simulink model "Es2_simulink"  (R2023a)
settings: Solver=VariableStepAuto  StartTime=0.0  StopTime=30  RelTol=1e-3
undefined symbols (not defined in the file or in its folder): ES2_emg, fdesignblkfcn, gcbh
libraries: dspfdesign x4, vrlib x1
settings Model: Creator=pisy1  LastModifiedBy=pisy1

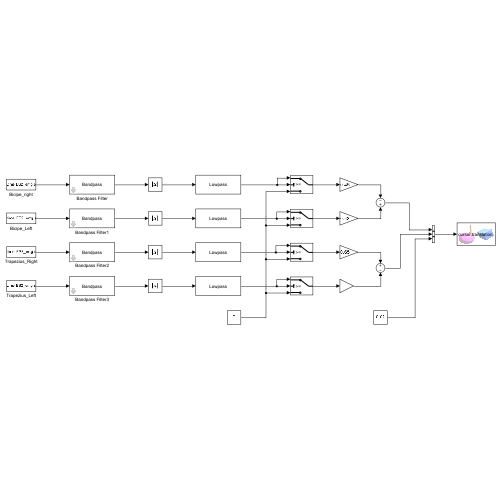
[thumbnail: Simulink's stored preview of the top-level diagram]
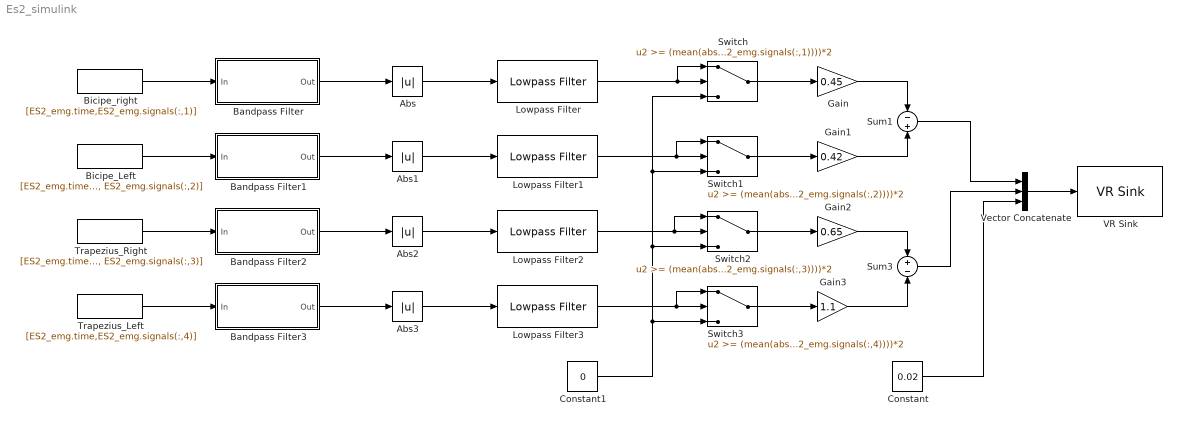
== system Es2_simulink ==
  Abs{,1..3} (4 alike) : Abs  SaturateOnIntegerOverflow=off
  Bandpass Filter : Subsystem  DialogController=fdesignblkfcn  InitFcn=fdesignblkfcn(gcbh, {'InitFcn'});  mask(Bandpass Filter){}
      mask help: dsp:DSPFilterDesignBlockDialog:BandpassFdesign_MaskDesc
      settings: CopyFcn=fdesignblkfcn(gcbh, {'CopyFcn'});
      mask Help: helpview(mapfilelocation('dsp'), 'dspbandpassfilter');
      mask Display: disp('Bandpass');
  Bandpass Filter1 : Subsystem  DialogController=fdesignblkfcn  InitFcn=fdesignblkfcn(gcbh, {'InitFcn'});  mask(Bandpass Filter){}
      mask help: dsp:DSPFilterDesignBlockDialog:BandpassFdesign_MaskDesc
      settings: CopyFcn=fdesignblkfcn(gcbh, {'CopyFcn'});
      mask Help: helpview(mapfilelocation('dsp'), 'dspbandpassfilter');
      mask Display: disp('Bandpass');
  Bandpass Filter2 : Subsystem  DialogController=fdesignblkfcn  InitFcn=fdesignblkfcn(gcbh, {'InitFcn'});  mask(Bandpass Filter){}
      mask help: dsp:DSPFilterDesignBlockDialog:BandpassFdesign_MaskDesc
      settings: CopyFcn=fdesignblkfcn(gcbh, {'CopyFcn'});
      mask Help: helpview(mapfilelocation('dsp'), 'dspbandpassfilter');
      mask Display: disp('Bandpass');
  Bandpass Filter3 : Subsystem  DialogController=fdesignblkfcn  InitFcn=fdesignblkfcn(gcbh, {'InitFcn'});  mask(Bandpass Filter){}
      mask help: dsp:DSPFilterDesignBlockDialog:BandpassFdesign_MaskDesc
      settings: CopyFcn=fdesignblkfcn(gcbh, {'CopyFcn'});
      mask Help: helpview(mapfilelocation('dsp'), 'dspbandpassfilter');
      mask Display: disp('Bandpass');
  Bicipe_Left : FromWorkspace  VariableName=[ES2_emg.time, ES2_emg.signals(:,2)]  SampleTime=1/1000
  Bicipe_right : FromWorkspace  VariableName=[ES2_emg.time,ES2_emg.signals(:,1)]  SampleTime=1/1000
  Constant : Constant  Value=0.02
  Constant1 : Constant  Value=0
  Gain : Gain  Gain=0.45
  Gain1 : Gain  Gain=0.42
  Gain2 : Gain  Gain=0.65
  Gain3 : Gain  Gain=1.1
  Lowpass Filter{,1..3} (4 alike) : dspfdesign/Lowpass Filter  FilterType=FIR  DesignForMinimumOrder=on  FilterOrder=50  PassbandFrequency=3  StopbandFrequency=6  PassbandRipple=0.1  StopbandAttenuation=80  SampleRateMode=Specify on dialog  SampleRate=1000  SimulateUsing=Interpreted execution  roundingMode=Floor  coeffsDataTypeStr=fixdt(1,16)
  Sum1 : Sum  Inputs=-|+
  Sum3 : Sum  Inputs=+|-
  Switch : Switch  Threshold=(mean(abs(ES2_emg.signals(:,1))))*2  SaturateOnIntegerOverflow=off  InputSameDT=off
  Switch1 : Switch  Threshold=(mean(abs(ES2_emg.signals(:,2))))*2  SaturateOnIntegerOverflow=off  InputSameDT=off
  Switch2 : Switch  Threshold=(mean(abs(ES2_emg.signals(:,3))))*2  SaturateOnIntegerOverflow=off  InputSameDT=off
  Switch3 : Switch  Threshold=(mean(abs(ES2_emg.signals(:,4))))*2  SaturateOnIntegerOverflow=off  InputSameDT=off
  Trapezius_Left : FromWorkspace  VariableName=[ES2_emg.time,ES2_emg.signals(:,4)]  SampleTime=1/1000
  Trapezius_Right : FromWorkspace  VariableName=[ES2_emg.time, ES2_emg.signals(:,3)]  SampleTime=1/1000
  VR Sink : vrlib/VR Sink  InstantiateOnLoad=on  SampleTime=0.1  ViewEnable=on  RemoteChange=off  RemoteView=off  FieldsWritten=cursor.translation.3.1.1.double  WorldFileName=8_palline_color.wrl  AutoView=off  VideoDimensions=[]  AllowVariableSize=off
  Vector Concatenate : Concatenate  NumInputs=3
  wires:
  Bandpass Filter/1(Out) -> Abs/1
  Abs/1 -> Lowpass Filter/1
  Abs1/1 -> Lowpass Filter1/1
  Abs2/1 -> Lowpass Filter2/1
  Abs3/1 -> Lowpass Filter3/1
  Bandpass Filter3/1(Out) -> Abs3/1
  Bandpass Filter2/1(Out) -> Abs2/1
  Bandpass Filter1/1(Out) -> Abs1/1
  Constant/1 -> Vector Concatenate/3
  Constant1/1 -> Switch/3, Switch1/3, Switch2/3, Switch3/3
  Lowpass Filter/1 -> Switch/1, Switch/2
  Lowpass Filter1/1 -> Switch1/1, Switch1/2
  Lowpass Filter2/1 -> Switch2/1, Switch2/2
  Lowpass Filter3/1 -> Switch3/1, Switch3/2
  Vector Concatenate/1 -> VR Sink/1
  Sum1/1 -> Vector Concatenate/1
  Sum3/1 -> Vector Concatenate/2
  Switch3/1 -> Gain3/1
  Switch2/1 -> Gain2/1
  Switch1/1 -> Gain1/1
  Switch/1 -> Gain/1
  Bicipe_Left/1 -> Bandpass Filter1/1(In)
  Bicipe_right/1 -> Bandpass Filter/1(In)
  Trapezius_Left/1 -> Bandpass Filter3/1(In)
  Trapezius_Right/1 -> Bandpass Filter2/1(In)
  Gain/1 -> Sum1/1
  Gain3/1 -> Sum3/2
  Gain2/1 -> Sum3/1
  Gain1/1 -> Sum1/2

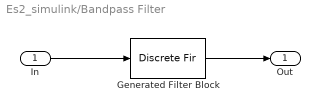
== system Es2_simulink/Bandpass Filter ==
  In : Inport
  Generated Filter Block : DiscreteFir  Tag=BlockMethodSubSystem  Coefficients=[-0.00268732969538467564 -0.0118693634414288839 -0.00464956295920984381 0.0192244660845699369 0.00401606132782830055 0.00113331359240486512 0.0081600274662763702 -0.00337347421316901196 0.00485232718819333594 -0.00260504936894014657 0.000574747267355126337 -0.00105940036214936546 -0.00260380481464203214 -1.31551187216019314e-05 -0.00436007271689453288 0.000301810052777536694 -0.00481839310143463047 -4.27651908615003795e-05 -0.00419699330761031525 -0.000850466496812417837 -0.002776431768186669 -0.00183710618674402196 -0.000931746391162900471 -0.00263535219191951726 0.000919518489321216603 -0.00287750193371332213 0.00234181011288215127 -0.0022885925310662655 0.00303033934142757019 -0.000818319173867537199 0.00290108759067781666 0.00132279014325093619 0.00211108519395160864 0.00367085202435546605 0.00104360943564956506 0.00558442951144205377 0.000169105346465872608 0.00645654583445923191 -0.000119621272358262989 0.00588287758558112082 0.000336400896954254514 0.00385123203778863117 0.00136139168005587272 0.000749506211944570011 0.00246191925777084104 -0.00266439972783858933 0.00298201898694502344 -0.0055265059231050977 0.00236131888729237136 -0.00708353416263684393 0.00033450104078665624 -0.00696088627834120025 -0.00288568812972243328 -0.0052797356224147194 -0.0065775442931197952 -0.00268218418692768058 -0.00964697208745706782 -7.2233731547276421e-05 -0.0109531527675894441 0.0016467062272919929 -0.00970504643296686217 0.00193564453488831792 -0.00571167618718560616 0.000850667168220128195 0.000409739809056720167 -0.000946605415802572597 0.00733164384418515808 -0.00232570671431918917 0.0133293503468598154 -0.00208261382497140855 0.0167413845912259031 0.000543802062682958998 0.0165183040724974223 0.00555728090932838467 0.0126095283934480155 0.0119157946244619097 0.00590275310015039509 0.0176861788427832844 -0.00170987438306957965 0.0205602710112455442 -0.0080752621768838441 0.0182809523079280126 -0.0113873648721023804 0.00965729454439472057 -0.0108374323953576782 -0.00513335134094568962 -0.00697642486247677246 -0.0240941247073598527 -0.00194247899233986054 -0.0437115227268439765 0.000972484332068239681 -0.0593855417670438313 -0.00220178639407756643 -0.0661386206551100586 -0.0155029767222636811 -0.0588085413080414038 -0.0436952688973444303 -0.0302190186977819297 -0.0973608444785738353 0.0433085287546407308 -0.244561056960632628 0.576859281938552626 0.576859281938552626 -0.244561056960632628 0.0433085287546407308 -0.0973608444785738353 -0.0302190186977819297 -0.0436952688973444303 -0.0588085413080414038 -0.0155029767222636811 -0.0661386206551100586 -0.00220178639407756643 -0.0593855417670438313 0.000972484332068239681 -0.0437115227268439765 -0.00194247899233986054 -0.0240941247073598527 -0.00697642486247677246 -0.00513335134094568962 -0.0108374323953576782 0.00965729454439472057 -0.0113873648721023804 0.0182809523079280126 -0.0080752621768838441 0.0205602710112455442 -0.00170987438306957965 0.0176861788427832844 0.00590275310015039509 0.0119157946244619097 0.0126095283934480155 0.00555728090932838467 0.0165183040724974223 0.000543802062682958998 0.0167413845912259031 -0.00208261382497140855 0.0133293503468598154 -0.00232570671431918917 0.00733164384418515808 -0.000946605415802572597 0.000409739809056720167 0.000850667168220128195 -0.00571167618718560616 0.00193564453488831792 -0.00970504643296686217 0.0016467062272919929 -0.0109531527675894441 -7.2233731547276421e-05 -0.00964697208745706782 -0.00268218418692768058 -0.0065775442931197952 -0.0052797356224147194 -0.00288568812972243328 -0.00696088627834120025 0.00033450104078665624 -0.00708353416263684393 0.00236131888729237136 -0.0055265059231050977 0.00298201898694502344 -0.00266439972783858933 0.00246191925777084104 0.000749506211944570011 0.00136139168005587272 0.00385123203778863117 0.000336400896954254514 0.00588287758558112082 -0.000119621272358262989 0.00645654583445923191 0.000169105346465872608 0.00558442951144205377 0.00104360943564956506 0.00367085202435546605 ...(+781 chars)]  InputProcessing=Columns as channels (frame based)
  Out : Outport  VectorParamsAs1DForOutWhenUnconnected=off
  wires:
  In/1 -> Generated Filter Block/1
  Generated Filter Block/1 -> Out/1

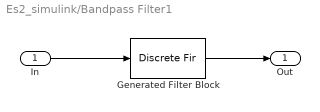
== system Es2_simulink/Bandpass Filter1 ==
  In : Inport
  Generated Filter Block : DiscreteFir  Tag=BlockMethodSubSystem  Coefficients=[-0.00268732969538467564 -0.0118693634414288839 -0.00464956295920984381 0.0192244660845699369 0.00401606132782830055 0.00113331359240486512 0.0081600274662763702 -0.00337347421316901196 0.00485232718819333594 -0.00260504936894014657 0.000574747267355126337 -0.00105940036214936546 -0.00260380481464203214 -1.31551187216019314e-05 -0.00436007271689453288 0.000301810052777536694 -0.00481839310143463047 -4.27651908615003795e-05 -0.00419699330761031525 -0.000850466496812417837 -0.002776431768186669 -0.00183710618674402196 -0.000931746391162900471 -0.00263535219191951726 0.000919518489321216603 -0.00287750193371332213 0.00234181011288215127 -0.0022885925310662655 0.00303033934142757019 -0.000818319173867537199 0.00290108759067781666 0.00132279014325093619 0.00211108519395160864 0.00367085202435546605 0.00104360943564956506 0.00558442951144205377 0.000169105346465872608 0.00645654583445923191 -0.000119621272358262989 0.00588287758558112082 0.000336400896954254514 0.00385123203778863117 0.00136139168005587272 0.000749506211944570011 0.00246191925777084104 -0.00266439972783858933 0.00298201898694502344 -0.0055265059231050977 0.00236131888729237136 -0.00708353416263684393 0.00033450104078665624 -0.00696088627834120025 -0.00288568812972243328 -0.0052797356224147194 -0.0065775442931197952 -0.00268218418692768058 -0.00964697208745706782 -7.2233731547276421e-05 -0.0109531527675894441 0.0016467062272919929 -0.00970504643296686217 0.00193564453488831792 -0.00571167618718560616 0.000850667168220128195 0.000409739809056720167 -0.000946605415802572597 0.00733164384418515808 -0.00232570671431918917 0.0133293503468598154 -0.00208261382497140855 0.0167413845912259031 0.000543802062682958998 0.0165183040724974223 0.00555728090932838467 0.0126095283934480155 0.0119157946244619097 0.00590275310015039509 0.0176861788427832844 -0.00170987438306957965 0.0205602710112455442 -0.0080752621768838441 0.0182809523079280126 -0.0113873648721023804 0.00965729454439472057 -0.0108374323953576782 -0.00513335134094568962 -0.00697642486247677246 -0.0240941247073598527 -0.00194247899233986054 -0.0437115227268439765 0.000972484332068239681 -0.0593855417670438313 -0.00220178639407756643 -0.0661386206551100586 -0.0155029767222636811 -0.0588085413080414038 -0.0436952688973444303 -0.0302190186977819297 -0.0973608444785738353 0.0433085287546407308 -0.244561056960632628 0.576859281938552626 0.576859281938552626 -0.244561056960632628 0.0433085287546407308 -0.0973608444785738353 -0.0302190186977819297 -0.0436952688973444303 -0.0588085413080414038 -0.0155029767222636811 -0.0661386206551100586 -0.00220178639407756643 -0.0593855417670438313 0.000972484332068239681 -0.0437115227268439765 -0.00194247899233986054 -0.0240941247073598527 -0.00697642486247677246 -0.00513335134094568962 -0.0108374323953576782 0.00965729454439472057 -0.0113873648721023804 0.0182809523079280126 -0.0080752621768838441 0.0205602710112455442 -0.00170987438306957965 0.0176861788427832844 0.00590275310015039509 0.0119157946244619097 0.0126095283934480155 0.00555728090932838467 0.0165183040724974223 0.000543802062682958998 0.0167413845912259031 -0.00208261382497140855 0.0133293503468598154 -0.00232570671431918917 0.00733164384418515808 -0.000946605415802572597 0.000409739809056720167 0.000850667168220128195 -0.00571167618718560616 0.00193564453488831792 -0.00970504643296686217 0.0016467062272919929 -0.0109531527675894441 -7.2233731547276421e-05 -0.00964697208745706782 -0.00268218418692768058 -0.0065775442931197952 -0.0052797356224147194 -0.00288568812972243328 -0.00696088627834120025 0.00033450104078665624 -0.00708353416263684393 0.00236131888729237136 -0.0055265059231050977 0.00298201898694502344 -0.00266439972783858933 0.00246191925777084104 0.000749506211944570011 0.00136139168005587272 0.00385123203778863117 0.000336400896954254514 0.00588287758558112082 -0.000119621272358262989 0.00645654583445923191 0.000169105346465872608 0.00558442951144205377 0.00104360943564956506 0.00367085202435546605 ...(+781 chars)]  InputProcessing=Columns as channels (frame based)
  Out : Outport  VectorParamsAs1DForOutWhenUnconnected=off
  wires:
  In/1 -> Generated Filter Block/1
  Generated Filter Block/1 -> Out/1

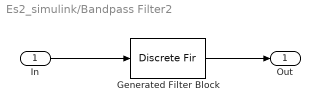
== system Es2_simulink/Bandpass Filter2 ==
  In : Inport
  Generated Filter Block : DiscreteFir  Tag=BlockMethodSubSystem  Coefficients=[-0.00268732969538467564 -0.0118693634414288839 -0.00464956295920984381 0.0192244660845699369 0.00401606132782830055 0.00113331359240486512 0.0081600274662763702 -0.00337347421316901196 0.00485232718819333594 -0.00260504936894014657 0.000574747267355126337 -0.00105940036214936546 -0.00260380481464203214 -1.31551187216019314e-05 -0.00436007271689453288 0.000301810052777536694 -0.00481839310143463047 -4.27651908615003795e-05 -0.00419699330761031525 -0.000850466496812417837 -0.002776431768186669 -0.00183710618674402196 -0.000931746391162900471 -0.00263535219191951726 0.000919518489321216603 -0.00287750193371332213 0.00234181011288215127 -0.0022885925310662655 0.00303033934142757019 -0.000818319173867537199 0.00290108759067781666 0.00132279014325093619 0.00211108519395160864 0.00367085202435546605 0.00104360943564956506 0.00558442951144205377 0.000169105346465872608 0.00645654583445923191 -0.000119621272358262989 0.00588287758558112082 0.000336400896954254514 0.00385123203778863117 0.00136139168005587272 0.000749506211944570011 0.00246191925777084104 -0.00266439972783858933 0.00298201898694502344 -0.0055265059231050977 0.00236131888729237136 -0.00708353416263684393 0.00033450104078665624 -0.00696088627834120025 -0.00288568812972243328 -0.0052797356224147194 -0.0065775442931197952 -0.00268218418692768058 -0.00964697208745706782 -7.2233731547276421e-05 -0.0109531527675894441 0.0016467062272919929 -0.00970504643296686217 0.00193564453488831792 -0.00571167618718560616 0.000850667168220128195 0.000409739809056720167 -0.000946605415802572597 0.00733164384418515808 -0.00232570671431918917 0.0133293503468598154 -0.00208261382497140855 0.0167413845912259031 0.000543802062682958998 0.0165183040724974223 0.00555728090932838467 0.0126095283934480155 0.0119157946244619097 0.00590275310015039509 0.0176861788427832844 -0.00170987438306957965 0.0205602710112455442 -0.0080752621768838441 0.0182809523079280126 -0.0113873648721023804 0.00965729454439472057 -0.0108374323953576782 -0.00513335134094568962 -0.00697642486247677246 -0.0240941247073598527 -0.00194247899233986054 -0.0437115227268439765 0.000972484332068239681 -0.0593855417670438313 -0.00220178639407756643 -0.0661386206551100586 -0.0155029767222636811 -0.0588085413080414038 -0.0436952688973444303 -0.0302190186977819297 -0.0973608444785738353 0.0433085287546407308 -0.244561056960632628 0.576859281938552626 0.576859281938552626 -0.244561056960632628 0.0433085287546407308 -0.0973608444785738353 -0.0302190186977819297 -0.0436952688973444303 -0.0588085413080414038 -0.0155029767222636811 -0.0661386206551100586 -0.00220178639407756643 -0.0593855417670438313 0.000972484332068239681 -0.0437115227268439765 -0.00194247899233986054 -0.0240941247073598527 -0.00697642486247677246 -0.00513335134094568962 -0.0108374323953576782 0.00965729454439472057 -0.0113873648721023804 0.0182809523079280126 -0.0080752621768838441 0.0205602710112455442 -0.00170987438306957965 0.0176861788427832844 0.00590275310015039509 0.0119157946244619097 0.0126095283934480155 0.00555728090932838467 0.0165183040724974223 0.000543802062682958998 0.0167413845912259031 -0.00208261382497140855 0.0133293503468598154 -0.00232570671431918917 0.00733164384418515808 -0.000946605415802572597 0.000409739809056720167 0.000850667168220128195 -0.00571167618718560616 0.00193564453488831792 -0.00970504643296686217 0.0016467062272919929 -0.0109531527675894441 -7.2233731547276421e-05 -0.00964697208745706782 -0.00268218418692768058 -0.0065775442931197952 -0.0052797356224147194 -0.00288568812972243328 -0.00696088627834120025 0.00033450104078665624 -0.00708353416263684393 0.00236131888729237136 -0.0055265059231050977 0.00298201898694502344 -0.00266439972783858933 0.00246191925777084104 0.000749506211944570011 0.00136139168005587272 0.00385123203778863117 0.000336400896954254514 0.00588287758558112082 -0.000119621272358262989 0.00645654583445923191 0.000169105346465872608 0.00558442951144205377 0.00104360943564956506 0.00367085202435546605 ...(+781 chars)]  InputProcessing=Columns as channels (frame based)
  Out : Outport  VectorParamsAs1DForOutWhenUnconnected=off
  wires:
  In/1 -> Generated Filter Block/1
  Generated Filter Block/1 -> Out/1

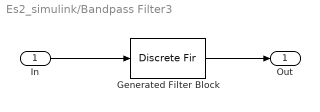
== system Es2_simulink/Bandpass Filter3 ==
  In : Inport
  Generated Filter Block : DiscreteFir  Tag=BlockMethodSubSystem  Coefficients=[-0.00268732969538467564 -0.0118693634414288839 -0.00464956295920984381 0.0192244660845699369 0.00401606132782830055 0.00113331359240486512 0.0081600274662763702 -0.00337347421316901196 0.00485232718819333594 -0.00260504936894014657 0.000574747267355126337 -0.00105940036214936546 -0.00260380481464203214 -1.31551187216019314e-05 -0.00436007271689453288 0.000301810052777536694 -0.00481839310143463047 -4.27651908615003795e-05 -0.00419699330761031525 -0.000850466496812417837 -0.002776431768186669 -0.00183710618674402196 -0.000931746391162900471 -0.00263535219191951726 0.000919518489321216603 -0.00287750193371332213 0.00234181011288215127 -0.0022885925310662655 0.00303033934142757019 -0.000818319173867537199 0.00290108759067781666 0.00132279014325093619 0.00211108519395160864 0.00367085202435546605 0.00104360943564956506 0.00558442951144205377 0.000169105346465872608 0.00645654583445923191 -0.000119621272358262989 0.00588287758558112082 0.000336400896954254514 0.00385123203778863117 0.00136139168005587272 0.000749506211944570011 0.00246191925777084104 -0.00266439972783858933 0.00298201898694502344 -0.0055265059231050977 0.00236131888729237136 -0.00708353416263684393 0.00033450104078665624 -0.00696088627834120025 -0.00288568812972243328 -0.0052797356224147194 -0.0065775442931197952 -0.00268218418692768058 -0.00964697208745706782 -7.2233731547276421e-05 -0.0109531527675894441 0.0016467062272919929 -0.00970504643296686217 0.00193564453488831792 -0.00571167618718560616 0.000850667168220128195 0.000409739809056720167 -0.000946605415802572597 0.00733164384418515808 -0.00232570671431918917 0.0133293503468598154 -0.00208261382497140855 0.0167413845912259031 0.000543802062682958998 0.0165183040724974223 0.00555728090932838467 0.0126095283934480155 0.0119157946244619097 0.00590275310015039509 0.0176861788427832844 -0.00170987438306957965 0.0205602710112455442 -0.0080752621768838441 0.0182809523079280126 -0.0113873648721023804 0.00965729454439472057 -0.0108374323953576782 -0.00513335134094568962 -0.00697642486247677246 -0.0240941247073598527 -0.00194247899233986054 -0.0437115227268439765 0.000972484332068239681 -0.0593855417670438313 -0.00220178639407756643 -0.0661386206551100586 -0.0155029767222636811 -0.0588085413080414038 -0.0436952688973444303 -0.0302190186977819297 -0.0973608444785738353 0.0433085287546407308 -0.244561056960632628 0.576859281938552626 0.576859281938552626 -0.244561056960632628 0.0433085287546407308 -0.0973608444785738353 -0.0302190186977819297 -0.0436952688973444303 -0.0588085413080414038 -0.0155029767222636811 -0.0661386206551100586 -0.00220178639407756643 -0.0593855417670438313 0.000972484332068239681 -0.0437115227268439765 -0.00194247899233986054 -0.0240941247073598527 -0.00697642486247677246 -0.00513335134094568962 -0.0108374323953576782 0.00965729454439472057 -0.0113873648721023804 0.0182809523079280126 -0.0080752621768838441 0.0205602710112455442 -0.00170987438306957965 0.0176861788427832844 0.00590275310015039509 0.0119157946244619097 0.0126095283934480155 0.00555728090932838467 0.0165183040724974223 0.000543802062682958998 0.0167413845912259031 -0.00208261382497140855 0.0133293503468598154 -0.00232570671431918917 0.00733164384418515808 -0.000946605415802572597 0.000409739809056720167 0.000850667168220128195 -0.00571167618718560616 0.00193564453488831792 -0.00970504643296686217 0.0016467062272919929 -0.0109531527675894441 -7.2233731547276421e-05 -0.00964697208745706782 -0.00268218418692768058 -0.0065775442931197952 -0.0052797356224147194 -0.00288568812972243328 -0.00696088627834120025 0.00033450104078665624 -0.00708353416263684393 0.00236131888729237136 -0.0055265059231050977 0.00298201898694502344 -0.00266439972783858933 0.00246191925777084104 0.000749506211944570011 0.00136139168005587272 0.00385123203778863117 0.000336400896954254514 0.00588287758558112082 -0.000119621272358262989 0.00645654583445923191 0.000169105346465872608 0.00558442951144205377 0.00104360943564956506 0.00367085202435546605 ...(+781 chars)]  InputProcessing=Columns as channels (frame based)
  Out : Outport  VectorParamsAs1DForOutWhenUnconnected=off
  wires:
  In/1 -> Generated Filter Block/1
  Generated Filter Block/1 -> Out/1
